simulink model "snap2_f_200msps_64i_4096c"  (R2019a)
settings: Solver=VariableStepDiscrete  StartTime=0.0  StopTime=10.0  RelTol=1e-3
undefined symbols (not defined in the file or in its folder): datetime, posixtime
libraries: xbsIndex_r4 x21354, casper_library_misc x297, casper_library_delays x19, xps_library x14, casper_library_sources x4
(part 4 of 217)

== system snap2_f_200msps_64i_4096c/delay ==
  note: counter starts at 1!!!
      | Simulation confirms this is the right
      | timing for the Serial -> Parallel converter to do The Right Thing
  sync : Inport
  din : Inport  Port=2
  65 : Subsystem  Commented=on
  Constant : xbsIndex_r4/Constant  const=2^max_delay_bits  gui_display_data_type=Fixed-point  arith_type=Unsigned  n_bits=32  bin_pt=0  preci_type=Single  exp_width=8  frac_width=24  explicit_period=on  period=1  equ=P=C  opselect=C  inp2=PCIN>>17  opr=+  inp1=P  carry=CIN  dbl_ovrd=off  block_type=constant
  Constant1 : xbsIndex_r4/Constant  Commented=on  const=0  gui_display_data_type=Fixed-point  arith_type=Unsigned  n_bits=32  bin_pt=0  preci_type=Single  exp_width=8  frac_width=24  explicit_period=on  period=1  equ=P=C  opselect=C  inp2=PCIN>>17  opr=+  inp1=P  carry=CIN  dbl_ovrd=off  block_type=constant
  Constant2 : xbsIndex_r4/Constant  Commented=on  const=0  gui_display_data_type=Boolean  arith_type=Boolean  n_bits=32  bin_pt=0  preci_type=Single  exp_width=8  frac_width=24  explicit_period=on  period=1  equ=P=C  opselect=C  inp2=PCIN>>17  opr=+  inp1=P  carry=CIN  dbl_ovrd=off  block_type=constant
  Counter : xbsIndex_r4/Counter  Commented=on  cnt_type=Free Running  cnt_to=Inf  operation=Up  start_count=1  cnt_by_val=1  arith_type=Unsigned  n_bits=6  bin_pt=0  load_pin=off  rst=off  en=off  explicit_period=on  period=1  use_behavioral_HDL=off  implementation=Fabric  dbl_ovrd=off  block_type=counter
  Delay : xbsIndex_r4/Delay  rst=off  infoeditControl=Selection of Reset will increase slice count due to use of real FFs and instead of SRLs  en=off  latency=7  reg_retiming=on  dbl_ovrd=off  block_type=delay
  Gateway Out{,1..7} (8 alike) : xbsIndex_r4/Gateway Out  Commented=on  inherit_from_input=off  hdl_port=off  rows=1  columns=1  UseAsDAC=off  DACChannel='1'  interface=None  automatic_assignment=on  address_offset=hex2dec('00')  intf_name=''  intf_description=''  timing_constraint=None  locs_specified=off  LOCs={}  io_standard={}  block_type=gatewayout
  Scope{,1..7} (8 alike) : Scope  Commented=on
  Serial to Parallel : xbsIndex_r4/Serial to Parallel  Commented=on  input_order=Most Significant Word First  arith_type=Unsigned  output_bits=13*64  bin_pt=0  rst=off  en=off  latency=1  dbl_ovrd=off  block_type=s2p
      settings: infoedit=Groups of samples presented serially at the input become single samples presented at the output.
  Slice : xbsIndex_r4/Slice  Commented=on  nbits=13  boolean_output=off  mode=Lower Bit Location + Width  bit1=0  base1=MSB of Input  bit0=0  base0=LSB of Input  dbl_ovrd=off  block_type=slice
  Slice1 : xbsIndex_r4/Slice  Commented=on  nbits=13  boolean_output=off  mode=Lower Bit Location + Width  bit1=0  base1=MSB of Input  bit0=0  base0=LSB of Input  dbl_ovrd=off  block_type=slice
  Slice2 : xbsIndex_r4/Slice  Commented=on  nbits=13  boolean_output=off  mode=Lower Bit Location + Width  bit1=0  base1=MSB of Input  bit0=13  base0=LSB of Input  dbl_ovrd=off  block_type=slice
  Slice3 : xbsIndex_r4/Slice  Commented=on  nbits=13  boolean_output=off  mode=Lower Bit Location + Width  bit1=0  base1=MSB of Input  bit0=13*2  base0=LSB of Input  dbl_ovrd=off  block_type=slice
  Subsystem : Subsystem
  Up Sample : xbsIndex_r4/Up Sample  Commented=on  sample_ratio=64  copy_samples=on  en=off  latency=1  dbl_ovrd=off  block_type=usamp
  bus_create : Subsystem  AncestorBlock=casper_library_flow_control/bus_create  mask(bus_create){inputNum=64}
      mask prompts: inputNum "Number of inputs:"
      mask init:
      | bus_create_init(gcb,...
      |     'inputNum', inputNum);
  bus_expand : Subsystem  AncestorBlock=casper_library_flow_control/bus_expand  mask(bus_expand){mode=divisions of equal size, outputNum=8*8, outputWidth=10, outputBinaryPt=0, outputArithmeticType=0, show_format=off, outputToWorkspace=off, variablePrefix=out, outputToModelAsWell=on}
      mask prompts: outputNum "Number of outputs:"; outputWidth "Output width:"; outputBinaryPt "Output binary point position:"; outputArithmeticType "Output arithmetic type (ufix=0, fix=1, bool=2):"; show_format "Print format string?"; outputToWorkspace "Output to workspace?"; variablePrefix "Variable name prefix:"; outputToModelAsWell "Output to model as well?"
      mask help:
      | Expands a 'bus' made using a bus_create or Xilinx
      | concat block.
      | The input will be divided into the specified number
      | of outputs with the specified arithmetic types.
      | Divisions are made from most significant bit.
      mask init: same as snap2_f_200msps_64i_4096c/autocorr/bus_expand
      settings: AttributesFormatString=64 outputs
      mask TypeOptions mode: divisions of equal size | divisions of arbitrary size
      mask Callback mode: bus_expand_callback();
      mask Callback outputWidth: bus_expand_callback();
      mask Callback outputToWorkspace: bus_expand_callback();
  bus_expand1 : Subsystem  AncestorBlock=casper_library_flow_control/bus_expand  mask(bus_expand){mode=divisions of equal size, outputNum=32, outputWidth=1, outputBinaryPt=0, outputArithmeticType=2, show_format=off, outputToWorkspace=off, variablePrefix=out, outputToModelAsWell=on}
      mask prompts: outputNum "Number of outputs:"; outputWidth "Output width:"; outputBinaryPt "Output binary point position:"; outputArithmeticType "Output arithmetic type (ufix=0, fix=1, bool=2):"; show_format "Print format string?"; outputToWorkspace "Output to workspace?"; variablePrefix "Variable name prefix:"; outputToModelAsWell "Output to model as well?"
      mask help:
      | Expands a 'bus' made using a bus_create or Xilinx
      | concat block.
      | The input will be divided into the specified number
      | of outputs with the specified arithmetic types.
      | Divisions are made from most significant bit.
      mask init: same as snap2_f_200msps_64i_4096c/autocorr/bus_expand
      settings: AttributesFormatString=32 outputs
      mask TypeOptions mode: divisions of equal size | divisions of arbitrary size
      mask Callback mode: bus_expand_callback();
      mask Callback outputWidth: bus_expand_callback();
      mask Callback outputToWorkspace: bus_expand_callback();
  bus_expand2 : Subsystem  AncestorBlock=casper_library_flow_control/bus_expand  mask(bus_expand){mode=divisions of equal size, outputNum=32, outputWidth=1, outputBinaryPt=0, outputArithmeticType=2, show_format=off, outputToWorkspace=off, variablePrefix=out, outputToModelAsWell=on}
      mask prompts: outputNum "Number of outputs:"; outputWidth "Output width:"; outputBinaryPt "Output binary point position:"; outputArithmeticType "Output arithmetic type (ufix=0, fix=1, bool=2):"; show_format "Print format string?"; outputToWorkspace "Output to workspace?"; variablePrefix "Variable name prefix:"; outputToModelAsWell "Output to model as well?"
      mask help:
      | Expands a 'bus' made using a bus_create or Xilinx
      | concat block.
      | The input will be divided into the specified number
      | of outputs with the specified arithmetic types.
      | Divisions are made from most significant bit.
      mask init: same as snap2_f_200msps_64i_4096c/autocorr/bus_expand
      settings: AttributesFormatString=32 outputs
      mask TypeOptions mode: divisions of equal size | divisions of arbitrary size
      mask Callback mode: bus_expand_callback();
      mask Callback outputWidth: bus_expand_callback();
      mask Callback outputToWorkspace: bus_expand_callback();
  delay0 : Subsystem  Tag=xps:sw_reg  AncestorBlock=xps_library/Memory/software_register  mask(swreg){io_dir=From Processor, io_delay=0, init_val=0, sample_period=1, names=reg, bitwidths=13, bin_pts=0, arith_types=0, sim_port=on, show_format=on, desc_str=""}
      mask prompts: io_dir "I/O direction"; io_delay "I/O delay"; init_val "Initial Value"; sample_period "Sample period"; names "Bitfield names [msb...lsb]"; bitwidths "Bitfield widths"; bin_pts "Bitfield binary pts"; arith_types "Bitfield types, ufix=0, fix=1, bool=2"; sim_port "Provide sim input/output?"; show_format "Print format string?"; desc_str "Description"
      mask help: A 32-bit software-accessible register. Can be divided into bitfields of varying widths and types using the fields in the block mask.
      mask init:
      | swreg_init(gcb)
      settings: AttributesFormatString=1input:uf13.0 = 13 bits
      mask TypeOptions io_dir: To Processor | From Processor
      mask Callback io_dir:
      | mask_enables = get_param(gcb, 'MaskEnables');
      | mask_names = get_param(gcb, 'MaskNames');
      | if strcmp(get_param(gcb, 'io_dir'), 'To Processor'),
      |     mask_enables{ismember(mask_names, 'sample_period')} = 'off';
      | else
      |     mask_enables{ismember(mask_names, 'sample_period')} = 'on';
      | end
      | set_param(gcb, 'MaskEnables', mask_enables);
      mask DialogControl ParameterTabVar0 Prompt: Setup
  delay1 : Subsystem  Tag=xps:sw_reg  AncestorBlock=xps_library/Memory/software_register  mask(swreg){io_dir=From Processor, io_delay=0, init_val=0, sample_period=1, names=reg, bitwidths=13, bin_pts=0, arith_types=0, sim_port=on, show_format=on, desc_str=""}
      mask prompts: io_dir "I/O direction"; io_delay "I/O delay"; init_val "Initial Value"; sample_period "Sample period"; names "Bitfield names [msb...lsb]"; bitwidths "Bitfield widths"; bin_pts "Bitfield binary pts"; arith_types "Bitfield types, ufix=0, fix=1, bool=2"; sim_port "Provide sim input/output?"; show_format "Print format string?"; desc_str "Description"
      mask help: A 32-bit software-accessible register. Can be divided into bitfields of varying widths and types using the fields in the block mask.
      mask init:
      | swreg_init(gcb)
      settings: AttributesFormatString=1input:uf13.0 = 13 bits
      mask TypeOptions io_dir: To Processor | From Processor
      mask Callback io_dir:
      | mask_enables = get_param(gcb, 'MaskEnables');
      | mask_names = get_param(gcb, 'MaskNames');
      | if strcmp(get_param(gcb, 'io_dir'), 'To Processor'),
      |     mask_enables{ismember(mask_names, 'sample_period')} = 'off';
      | else
      |     mask_enables{ismember(mask_names, 'sample_period')} = 'on';
      | end
      | set_param(gcb, 'MaskEnables', mask_enables);
      mask DialogControl ParameterTabVar0 Prompt: Setup
  delay_en0 : Subsystem  Tag=xps:sw_reg  AncestorBlock=xps_library/Memory/software_register  mask(swreg){io_dir=From Processor, io_delay=0, init_val=0, sample_period=1, names=reg, bitwidths=32, bin_pts=0, arith_types=0, sim_port=on, show_format=on, desc_str=""}
      mask prompts: io_dir "I/O direction"; io_delay "I/O delay"; init_val "Initial Value"; sample_period "Sample period"; names "Bitfield names [msb...lsb]"; bitwidths "Bitfield widths"; bin_pts "Bitfield binary pts"; arith_types "Bitfield types, ufix=0, fix=1, bool=2"; sim_port "Provide sim input/output?"; show_format "Print format string?"; desc_str "Description"
      mask help: A 32-bit software-accessible register. Can be divided into bitfields of varying widths and types using the fields in the block mask.
      mask init:
      | swreg_init(gcb)
      settings: AttributesFormatString=1input:uf32.0 = 32 bits
      mask TypeOptions io_dir: To Processor | From Processor
      mask Callback io_dir:
      | mask_enables = get_param(gcb, 'MaskEnables');
      | mask_names = get_param(gcb, 'MaskNames');
      | if strcmp(get_param(gcb, 'io_dir'), 'To Processor'),
      |     mask_enables{ismember(mask_names, 'sample_period')} = 'off';
      | else
      |     mask_enables{ismember(mask_names, 'sample_period')} = 'on';
      | end
      | set_param(gcb, 'MaskEnables', mask_enables);
      mask DialogControl ParameterTabVar0 Prompt: Setup
  delay_en1 : Subsystem  Tag=xps:sw_reg  AncestorBlock=xps_library/Memory/software_register  mask(swreg){io_dir=From Processor, io_delay=0, init_val=0, sample_period=1, names=reg, bitwidths=32, bin_pts=0, arith_types=0, sim_port=on, show_format=on, desc_str=""}
      mask prompts: io_dir "I/O direction"; io_delay "I/O delay"; init_val "Initial Value"; sample_period "Sample period"; names "Bitfield names [msb...lsb]"; bitwidths "Bitfield widths"; bin_pts "Bitfield binary pts"; arith_types "Bitfield types, ufix=0, fix=1, bool=2"; sim_port "Provide sim input/output?"; show_format "Print format string?"; desc_str "Description"
      mask help: A 32-bit software-accessible register. Can be divided into bitfields of varying widths and types using the fields in the block mask.
      mask init:
      | swreg_init(gcb)
      settings: AttributesFormatString=1input:uf32.0 = 32 bits
      mask TypeOptions io_dir: To Processor | From Processor
      mask Callback io_dir:
      | mask_enables = get_param(gcb, 'MaskEnables');
      | mask_names = get_param(gcb, 'MaskNames');
      | if strcmp(get_param(gcb, 'io_dir'), 'To Processor'),
      |     mask_enables{ismember(mask_names, 'sample_period')} = 'off';
      | else
      |     mask_enables{ismember(mask_names, 'sample_period')} = 'on';
      | end
      | set_param(gcb, 'MaskEnables', mask_enables);
      mask DialogControl ParameterTabVar0 Prompt: Setup
  delay_store0 : Subsystem
  delay_store1 : Subsystem
  delays : Subsystem  Tag=xps:bram  Commented=on  AncestorBlock=xps_library/Memory/shared_bram  mask{sample_rate=1, init_vals=[0:2^6-1], data_bin_pt=0, optimization=Minimum_Area, reg_core_output=off, reg_prim_output=off, data_width=32, addr_width=6, arith_type=Unsigned, desc_str="", type_desc=""}
      mask prompts: sample_rate "Sample rate"; init_vals "Initial values (simulation only)"; data_bin_pt "Data Binary Point"; reg_core_output "Register Core Output"; reg_prim_output "Register Primitive Output"; data_width "Data Width"; addr_width "Address width"; arith_type "Output Data Type"; desc_str "Description"; type_desc "Word Type Description"
      mask init:
      | shared_bram_mask;
      mask TypeOptions optimization: Minimum_Area | Low_Power
      mask TypeOptions data_width: 8 | 16 | 32 | 64 | 128
      mask TypeOptions arith_type: Unsigned | Signed  (2's comp)
      mask DialogControl Container4 Prompt: Configuration
      mask DialogControl Container10 Prompt: Documentation
  max_delay : Subsystem  Tag=xps:sw_reg  AncestorBlock=xps_library/Memory/software_register  mask(swreg){io_dir=To Processor, io_delay=0, init_val=0, sample_period=1, names=reg, bitwidths=32, bin_pts=0, arith_types=0, sim_port=on, show_format=off, desc_str=|}
      mask desc_str=|
      | Interpretted as a unint32 value, contains the maximum
      | allowed delay, in ADC samples, which may be applied
      | to a data stream.
      mask prompts: io_dir "I/O direction"; io_delay "I/O delay"; init_val "Initial Value"; sample_period "Sample period"; names "Bitfield names [msb...lsb]"; bitwidths "Bitfield widths"; bin_pts "Bitfield binary pts"; arith_types "Bitfield types, ufix=0, fix=1, bool=2"; sim_port "Provide sim input/output?"; show_format "Print format string?"; desc_str "Description"
      mask help: A 32-bit software-accessible register. Can be divided into bitfields of varying widths and types using the fields in the block mask.
      mask init:
      | swreg_init(gcb)
      settings: AttributesFormatString=1output
      mask TypeOptions io_dir: To Processor | From Processor
      mask Callback io_dir:
      | mask_enables = get_param(gcb, 'MaskEnables');
      | mask_names = get_param(gcb, 'MaskNames');
      | if strcmp(get_param(gcb, 'io_dir'), 'To Processor'),
      |     mask_enables{ismember(mask_names, 'sample_period')} = 'off';
      | else
      |     mask_enables{ismember(mask_names, 'sample_period')} = 'on';
      | end
      | set_param(gcb, 'MaskEnables', mask_enables);
      mask DialogControl ParameterTabVar0 Prompt: Setup
  sync_out : Outport
  dout : Outport  Port=2
  wires:
  sync/1 -> Delay/1
  din/1 -> bus_expand/1(bus_in)
  bus_create/1(bus_out) -> dout/1
  Constant/1 -> max_delay/1(out_reg)
  Delay/1 -> sync_out/1
  Counter/1 -> delays/1(addr)
  Constant1/1 -> delays/2(data_in)
  Constant2/1 -> delays/3(we)
  delays/1(data_out) -> Slice/1
  Serial to Parallel/1 -> Up Sample/1, Slice3/1, Slice2/1, Slice1/1
  Slice/1 -> Gateway Out/1, Serial to Parallel/1
  Subsystem/1(Out1) -> bus_create/1(in1)
  Subsystem/2(Out2) -> bus_create/2(in2)
  Subsystem/3(Out3) -> bus_create/3(in3)
  Subsystem/4(Out4) -> bus_create/4(in4)
  Subsystem/5(Out5) -> bus_create/5(in5)
  Subsystem/6(Out6) -> bus_create/6(in6)
  Subsystem/7(Out7) -> bus_create/7(in7)
  Subsystem/8(Out8) -> bus_create/8(in8)
  Subsystem/9(Out9) -> bus_create/9(in9)
  Subsystem/10(Out10) -> bus_create/10(in10)
  Subsystem/11(Out11) -> bus_create/11(in11)
  Subsystem/12(Out12) -> bus_create/12(in12)
  Subsystem/13(Out13) -> bus_create/13(in13)
  Subsystem/14(Out14) -> bus_create/14(in14)
  Subsystem/15(Out15) -> bus_create/15(in15)
  Subsystem/16(Out16) -> bus_create/16(in16)
  Subsystem/17(Out17) -> bus_create/17(in17)
  Subsystem/18(Out18) -> bus_create/18(in18)
  Subsystem/19(Out19) -> bus_create/19(in19)
  Subsystem/20(Out20) -> bus_create/20(in20)
  Subsystem/21(Out21) -> bus_create/21(in21)
  Subsystem/22(Out22) -> bus_create/22(in22)
  Subsystem/23(Out23) -> bus_create/23(in23)
  Subsystem/24(Out24) -> bus_create/24(in24)
  Subsystem/25(Out25) -> bus_create/25(in25)
  Subsystem/26(Out26) -> bus_create/26(in26)
  Subsystem/27(Out27) -> bus_create/27(in27)
  Subsystem/28(Out28) -> bus_create/28(in28)
  Subsystem/29(Out29) -> bus_create/29(in29)
  Subsystem/30(Out30) -> bus_create/30(in30)
  Subsystem/31(Out31) -> bus_create/31(in31)
  Subsystem/32(Out32) -> bus_create/32(in32)
  Subsystem/33(Out33) -> bus_create/33(in33)
  Subsystem/34(Out34) -> bus_create/34(in34)
  Subsystem/35(Out35) -> bus_create/35(in35)
  Subsystem/36(Out36) -> bus_create/36(in36)
  Subsystem/37(Out37) -> bus_create/37(in37)
  Subsystem/38(Out38) -> bus_create/38(in38)
  Subsystem/39(Out39) -> bus_create/39(in39)
  Subsystem/40(Out40) -> bus_create/40(in40)
  Subsystem/41(Out41) -> bus_create/41(in41)
  Subsystem/42(Out42) -> bus_create/42(in42)
  Subsystem/43(Out43) -> bus_create/43(in43)
  Subsystem/44(Out44) -> bus_create/44(in44)
  Subsystem/45(Out45) -> bus_create/45(in45)
  Subsystem/46(Out46) -> bus_create/46(in46)
  Subsystem/47(Out47) -> bus_create/47(in47)
  Subsystem/48(Out48) -> bus_create/48(in48)
  Subsystem/49(Out49) -> bus_create/49(in49)
  Subsystem/50(Out50) -> bus_create/50(in50)
  Subsystem/51(Out51) -> bus_create/51(in51)
  Subsystem/52(Out52) -> bus_create/52(in52)
  Subsystem/53(Out53) -> bus_create/53(in53)
  Subsystem/54(Out54) -> bus_create/54(in54)
  Subsystem/55(Out55) -> bus_create/55(in55)
  Subsystem/56(Out56) -> bus_create/56(in56)
  Subsystem/57(Out57) -> bus_create/57(in57)
  Subsystem/58(Out58) -> bus_create/58(in58)
  Subsystem/59(Out59) -> bus_create/59(in59)
  Subsystem/60(Out60) -> bus_create/60(in60)
  Subsystem/61(Out61) -> bus_create/61(in61)
  Subsystem/62(Out62) -> bus_create/62(in62)
  Subsystem/63(Out63) -> bus_create/63(in63)
  Subsystem/64(Out64) -> bus_create/64(in64)
  bus_expand/1(msb_out64) -> Subsystem/1(In1)
  bus_expand/2(out63) -> Subsystem/2(In3)
  bus_expand/3(out62) -> Subsystem/3(In2)
  bus_expand/4(out61) -> Subsystem/4(In4)
  bus_expand/5(out60) -> Subsystem/5(In5)
  bus_expand/6(out59) -> Subsystem/6(In6)
  bus_expand/7(out58) -> Subsystem/7(In7)
  bus_expand/8(out57) -> Subsystem/8(In8)
  bus_expand/9(out56) -> Subsystem/9(In9)
  bus_expand/10(out55) -> Subsystem/10(In10)
  bus_expand/11(out54) -> Subsystem/11(In11)
  bus_expand/12(out53) -> Subsystem/12(In12)
  bus_expand/13(out52) -> Subsystem/13(In13)
  bus_expand/14(out51) -> Subsystem/14(In14)
  bus_expand/15(out50) -> Subsystem/15(In15)
  bus_expand/16(out49) -> Subsystem/16(In16)
  bus_expand/17(out48) -> Subsystem/17(In17)
  bus_expand/18(out47) -> Subsystem/18(In18)
  bus_expand/19(out46) -> Subsystem/19(In19)
  bus_expand/20(out45) -> Subsystem/20(In20)
  bus_expand/21(out44) -> Subsystem/21(In21)
  bus_expand/22(out43) -> Subsystem/22(In22)
  bus_expand/23(out42) -> Subsystem/23(In23)
  bus_expand/24(out41) -> Subsystem/24(In24)
  bus_expand/25(out40) -> Subsystem/25(In25)
  bus_expand/26(out39) -> Subsystem/26(In26)
  bus_expand/27(out38) -> Subsystem/27(In27)
  bus_expand/28(out37) -> Subsystem/28(In28)
  bus_expand/29(out36) -> Subsystem/29(In29)
  bus_expand/30(out35) -> Subsystem/30(In30)
  bus_expand/31(out34) -> Subsystem/31(In31)
  bus_expand/32(out33) -> Subsystem/32(In32)
  bus_expand/33(out32) -> Subsystem/33(In33)
  bus_expand/34(out31) -> Subsystem/34(In34)
  bus_expand/35(out30) -> Subsystem/35(In35)
  bus_expand/36(out29) -> Subsystem/36(In36)
  bus_expand/37(out28) -> Subsystem/37(In37)
  bus_expand/38(out27) -> Subsystem/38(In38)
  bus_expand/39(out26) -> Subsystem/39(In39)
  bus_expand/40(out25) -> Subsystem/40(In40)
  bus_expand/41(out24) -> Subsystem/41(In41)
  bus_expand/42(out23) -> Subsystem/42(In42)
  bus_expand/43(out22) -> Subsystem/43(In43)
  bus_expand/44(out21) -> Subsystem/44(In44)
  bus_expand/45(out20) -> Subsystem/45(In45)
  bus_expand/46(out19) -> Subsystem/46(In46)
  bus_expand/47(out18) -> Subsystem/47(In47)
  bus_expand/48(out17) -> Subsystem/48(In48)
  bus_expand/49(out16) -> Subsystem/49(In49)
  bus_expand/50(out15) -> Subsystem/50(In50)
  bus_expand/51(out14) -> Subsystem/51(In51)
  bus_expand/52(out13) -> Subsystem/52(In52)
  bus_expand/53(out12) -> Subsystem/53(In53)
  bus_expand/54(out11) -> Subsystem/54(In54)
  bus_expand/55(out10) -> Subsystem/55(In55)
  bus_expand/56(out9) -> Subsystem/56(In56)
  bus_expand/57(out8) -> Subsystem/57(In57)
  bus_expand/58(out7) -> Subsystem/58(In58)
  bus_expand/59(out6) -> Subsystem/59(In59)
  bus_expand/60(out5) -> Subsystem/60(In60)
  bus_expand/61(out4) -> Subsystem/61(In61)
  bus_expand/62(out3) -> Subsystem/62(In62)
  bus_expand/63(out2) -> Subsystem/63(In63)
  bus_expand/64(lsb_out1) -> Subsystem/64(In64)
  Gateway Out/1 -> Scope/1
  Gateway Out1/1 -> Scope1/1
  Gateway Out2/1 -> Scope2/1
  Gateway Out3/1 -> Scope3/1
  Slice1/1 -> Gateway Out3/1
  Slice2/1 -> Gateway Out4/1
  Gateway Out4/1 -> Scope4/1
  Gateway Out5/1 -> Scope5/1
  Slice3/1 -> Gateway Out5/1
  Gateway Out7/1 -> Scope7/1
  Gateway Out6/1 -> Scope6/1
  delay0/1(in_reg) -> delay_store0/1(delay_in)
  delay_store0/1(delay0) -> Subsystem/65(delay1)
  delay_store0/2(delay1) -> Subsystem/66(delay2)
  delay_store0/3(delay2) -> Subsystem/67(delay3)
  delay_store0/4(delay3) -> Subsystem/68(delay4)
  delay_store0/5(delay4) -> Subsystem/69(delay5)
  delay_store0/6(delay5) -> Subsystem/70(delay6)
  delay_store0/7(delay6) -> Subsystem/71(delay7)
  delay_store0/8(delay7) -> Subsystem/72(delay8)
  delay_store0/9(delay8) -> Subsystem/73(delay9)
  delay_store0/10(delay9) -> Subsystem/74(delay10)
  delay_store0/11(delay10) -> Subsystem/75(delay11)
  delay_store0/12(delay11) -> Subsystem/76(delay12)
  delay_store0/13(delay12) -> Subsystem/77(delay13)
  delay_store0/14(delay13) -> Subsystem/78(delay14)
  delay_store0/15(delay14) -> Subsystem/79(delay15)
  delay_store0/16(delay15) -> Subsystem/80(delay16)
  delay_store0/17(delay16) -> Subsystem/81(delay17)
  delay_store0/18(delay17) -> Subsystem/82(delay18)
  delay_store0/19(delay18) -> Subsystem/83(delay19)
  delay_store0/20(delay19) -> Subsystem/84(delay20)
  delay_store0/21(delay20) -> Subsystem/85(delay21)
  delay_store0/22(delay21) -> Subsystem/86(delay22)
  delay_store0/23(delay22) -> Subsystem/87(delay23)
  delay_store0/24(delay23) -> Subsystem/88(delay24)
  delay_store0/25(delay24) -> Subsystem/89(delay25)
  delay_store0/26(delay25) -> Subsystem/90(delay26)
  delay_store0/27(delay26) -> Subsystem/91(delay27)
  delay_store0/28(delay27) -> Subsystem/92(delay28)
  delay_store0/29(delay28) -> Subsystem/93(delay29)
  delay_store0/30(delay29) -> Subsystem/94(delay30)
  delay_store0/31(delay30) -> Subsystem/95(delay31)
  delay_store0/32(delay31) -> Subsystem/96(delay32)
  delay_store1/1(delay0) -> Subsystem/97(delay33)
  delay_store1/2(delay1) -> Subsystem/98(delay34)
  delay_store1/3(delay2) -> Subsystem/99(delay35)
  delay_store1/4(delay3) -> Subsystem/100(delay36)
  delay_store1/5(delay4) -> Subsystem/101(delay37)
  delay_store1/6(delay5) -> Subsystem/102(delay38)
  delay_store1/7(delay6) -> Subsystem/103(delay39)
  delay_store1/8(delay7) -> Subsystem/104(delay40)
  delay_store1/9(delay8) -> Subsystem/105(delay41)
  delay_store1/10(delay9) -> Subsystem/106(delay42)
  delay_store1/11(delay10) -> Subsystem/107(delay43)
  delay_store1/12(delay11) -> Subsystem/108(delay44)
  delay_store1/13(delay12) -> Subsystem/109(delay45)
  delay_store1/14(delay13) -> Subsystem/110(delay46)
  delay_store1/15(delay14) -> Subsystem/111(delay47)
  delay_store1/16(delay15) -> Subsystem/112(delay48)
  delay_store1/17(delay16) -> Subsystem/113(delay49)
  delay_store1/18(delay17) -> Subsystem/114(delay50)
  delay_store1/19(delay18) -> Subsystem/115(delay51)
  delay_store1/20(delay19) -> Subsystem/116(delay52)
  delay_store1/21(delay20) -> Subsystem/117(delay53)
  delay_store1/22(delay21) -> Subsystem/118(delay54)
  delay_store1/23(delay22) -> Subsystem/119(delay55)
  delay_store1/24(delay23) -> Subsystem/120(delay56)
  delay_store1/25(delay24) -> Subsystem/121(delay57)
  delay_store1/26(delay25) -> Subsystem/122(delay58)
  delay_store1/27(delay26) -> Subsystem/123(delay59)
  delay_store1/28(delay27) -> Subsystem/124(delay60)
  delay_store1/29(delay28) -> Subsystem/125(delay61)
  delay_store1/30(delay29) -> Subsystem/126(delay62)
  delay_store1/31(delay30) -> Subsystem/127(delay63)
  delay_store1/32(delay31) -> Subsystem/128(delay64)
  bus_expand1/1(msb_out32) -> delay_store0/2(en0)
  bus_expand1/2(out31) -> delay_store0/3(en1)
  bus_expand1/3(out30) -> delay_store0/4(en2)
  bus_expand1/4(out29) -> delay_store0/5(en3)
  bus_expand1/5(out28) -> delay_store0/6(en4)
  bus_expand1/6(out27) -> delay_store0/7(en5)
  bus_expand1/7(out26) -> delay_store0/8(en6)
  bus_expand1/8(out25) -> delay_store0/9(en7)
  bus_expand1/9(out24) -> delay_store0/10(en8)
  bus_expand1/10(out23) -> delay_store0/11(en9)
  bus_expand1/11(out22) -> delay_store0/12(en10)
  bus_expand1/12(out21) -> delay_store0/13(en11)
  bus_expand1/13(out20) -> delay_store0/14(en12)
  bus_expand1/14(out19) -> delay_store0/15(en13)
  bus_expand1/15(out18) -> delay_store0/16(en14)
  bus_expand1/16(out17) -> delay_store0/17(en15)
  bus_expand1/17(out16) -> delay_store0/18(en16)
  bus_expand1/18(out15) -> delay_store0/19(en17)
  bus_expand1/19(out14) -> delay_store0/20(en18)
  bus_expand1/20(out13) -> delay_store0/21(en19)
  bus_expand1/21(out12) -> delay_store0/22(en20)
  bus_expand1/22(out11) -> delay_store0/23(en21)
  bus_expand1/23(out10) -> delay_store0/24(en22)
  bus_expand1/24(out9) -> delay_store0/25(en23)
  bus_expand1/25(out8) -> delay_store0/26(en24)
  bus_expand1/26(out7) -> delay_store0/27(en25)
  bus_expand1/27(out6) -> delay_store0/28(en26)
  bus_expand1/28(out5) -> delay_store0/29(en27)
  bus_expand1/29(out4) -> delay_store0/30(en28)
  bus_expand1/30(out3) -> delay_store0/31(en29)
  bus_expand1/31(out2) -> delay_store0/32(en30)
  bus_expand1/32(lsb_out1) -> delay_store0/33(en31)
  delay_en0/1(in_reg) -> bus_expand1/1(bus_in)
  delay_en1/1(in_reg) -> bus_expand2/1(bus_in)
  delay1/1(in_reg) -> delay_store1/1(delay_in)
  bus_expand2/1(msb_out32) -> delay_store1/2(en0)
  bus_expand2/2(out31) -> delay_store1/3(en1)
  bus_expand2/3(out30) -> delay_store1/4(en2)
  bus_expand2/4(out29) -> delay_store1/5(en3)
  bus_expand2/5(out28) -> delay_store1/6(en4)
  bus_expand2/6(out27) -> delay_store1/7(en5)
  bus_expand2/7(out26) -> delay_store1/8(en6)
  bus_expand2/8(out25) -> delay_store1/9(en7)
  bus_expand2/9(out24) -> delay_store1/10(en8)
  bus_expand2/10(out23) -> delay_store1/11(en9)
  bus_expand2/11(out22) -> delay_store1/12(en10)
  bus_expand2/12(out21) -> delay_store1/13(en11)
  bus_expand2/13(out20) -> delay_store1/14(en12)
  bus_expand2/14(out19) -> delay_store1/15(en13)
  bus_expand2/15(out18) -> delay_store1/16(en14)
  bus_expand2/16(out17) -> delay_store1/17(en15)
  bus_expand2/17(out16) -> delay_store1/18(en16)
  bus_expand2/18(out15) -> delay_store1/19(en17)
  bus_expand2/19(out14) -> delay_store1/20(en18)
  bus_expand2/20(out13) -> delay_store1/21(en19)
  bus_expand2/21(out12) -> delay_store1/22(en20)
  bus_expand2/22(out11) -> delay_store1/23(en21)
  bus_expand2/23(out10) -> delay_store1/24(en22)
  bus_expand2/24(out9) -> delay_store1/25(en23)
  bus_expand2/25(out8) -> delay_store1/26(en24)
  bus_expand2/26(out7) -> delay_store1/27(en25)
  bus_expand2/27(out6) -> delay_store1/28(en26)
  bus_expand2/28(out5) -> delay_store1/29(en27)
  bus_expand2/29(out4) -> delay_store1/30(en28)
  bus_expand2/30(out3) -> delay_store1/31(en29)
  bus_expand2/31(out2) -> delay_store1/32(en30)
  bus_expand2/32(lsb_out1) -> delay_store1/33(en31)

== system snap2_f_200msps_64i_4096c/eq ==
  sync : Inport
  din : Inport  Port=2
  bus_create2 : Subsystem  AncestorBlock=casper_library_flow_control/bus_create  mask(bus_create){inputNum=4}
      mask prompts: inputNum "Number of inputs:"
      mask init:
      | bus_create_init(gcb,...
      |     'inputNum', inputNum);
  bus_expand4 : Subsystem  AncestorBlock=casper_library_flow_control/bus_expand  mask(bus_expand){mode=divisions of equal size, outputNum=4, outputWidth=36*8, outputBinaryPt=0, outputArithmeticType=0, show_format=off, outputToWorkspace=off, variablePrefix=out, outputToModelAsWell=on}
      mask prompts: outputNum "Number of outputs:"; outputWidth "Output width:"; outputBinaryPt "Output binary point position:"; outputArithmeticType "Output arithmetic type (ufix=0, fix=1, bool=2):"; show_format "Print format string?"; outputToWorkspace "Output to workspace?"; variablePrefix "Variable name prefix:"; outputToModelAsWell "Output to model as well?"
      mask help:
      | Expands a 'bus' made using a bus_create or Xilinx
      | concat block.
      | The input will be divided into the specified number
      | of outputs with the specified arithmetic types.
      | Divisions are made from most significant bit.
      mask init: same as snap2_f_200msps_64i_4096c/autocorr/bus_expand
      settings: AttributesFormatString=4 outputs
      mask TypeOptions mode: divisions of equal size | divisions of arbitrary size
      mask Callback mode: bus_expand_callback();
      mask Callback outputWidth: bus_expand_callback();
      mask Callback outputToWorkspace: bus_expand_callback();
  core0 : Subsystem  mask{nchan=12-3, nants=16, n_bp=2}
      mask prompts: nchan "Number of fft channels (2^?)"; nants "Number of Antennas"; n_bp "Coefficient binary point position"
  core1 : Subsystem  mask{nchan=12-3, nants=16, n_bp=2}
      mask prompts: nchan "Number of fft channels (2^?)"; nants "Number of Antennas"; n_bp "Coefficient binary point position"
  core2 : Subsystem  mask{nchan=12-3, nants=16, n_bp=2}
      mask prompts: nchan "Number of fft channels (2^?)"; nants "Number of Antennas"; n_bp "Coefficient binary point position"
  core3 : Subsystem  mask{nchan=12-3, nants=16, n_bp=2}
      mask prompts: nchan "Number of fft channels (2^?)"; nants "Number of Antennas"; n_bp "Coefficient binary point position"
  sync_out : Outport
  dout : Outport  Port=2
  wires:
  core0/1(sync_out) -> sync_out/1
  din/1 -> bus_expand4/1(bus_in)
  sync/1 -> [sync_in]
  [sync_in] -> core0/1(sync)
  [sync_in] -> core1/1(sync)
  [sync_in] -> core2/1(sync)
  [sync_in] -> core3/1(sync)
  bus_expand4/1(msb_out4) -> core0/2(in)
  bus_expand4/2(out3) -> core1/2(in)
  bus_expand4/3(out2) -> core2/2(in)
  bus_expand4/4(lsb_out1) -> core3/2(in)
  core1/1(sync_out) -> ?
  core2/1(sync_out) -> ?
  core3/1(sync_out) -> ?
  core1/2(dout) -> bus_create2/2(in2)
  core2/2(dout) -> bus_create2/3(in3)
  core0/2(dout) -> bus_create2/1(in1)
  core3/2(dout) -> bus_create2/4(in4)
  bus_create2/1(bus_out) -> dout/1

== system snap2_f_200msps_64i_4096c/eth ==
  note: bit 19
  note: bit 18
  note: bit 1
  note: bit 0
  note: only allow enable
      | state to change at the end
      | of a packet.
      |
      | This avoids overflows arising
      | from part of a packet being
      | clocked in to the core
      | but the EOF being disable
  data : Inport
  vld : Inport  Port=2
  eof : Inport  Port=3
  dest_ip : Inport  Port=4
  port : Inport  Port=5
  Constant : xbsIndex_r4/Constant  const=0  gui_display_data_type=Boolean  arith_type=Boolean  n_bits=1  bin_pt=0  preci_type=Single  exp_width=8  frac_width=24  explicit_period=on  period=1  equ=P=C  opselect=C  inp2=PCIN>>17  opr=+  inp1=P  carry=CIN  dbl_ovrd=off  block_type=constant
  Constant1 : xbsIndex_r4/Constant  const=0  gui_display_data_type=Boolean  arith_type=Boolean  n_bits=1  bin_pt=0  preci_type=Single  exp_width=8  frac_width=24  explicit_period=on  period=1  equ=P=C  opselect=C  inp2=PCIN>>17  opr=+  inp1=P  carry=CIN  dbl_ovrd=off  block_type=constant
  Delay{5..11} (7 alike) : xbsIndex_r4/Delay  rst=off  infoeditControl=Selection of Reset will increase slice count due to use of real FFs and instead of SRLs  en=off  latency=1  reg_retiming=off  dbl_ovrd=off  block_type=delay
  Logical : xbsIndex_r4/Logical  logical_function=AND  inputs=2  en=off  latency=0  precision=Full  arith_type=Unsigned  n_bits=16  bin_pt=0  align_bp=on  dbl_ovrd=off  block_type=logical
  Logical1 : xbsIndex_r4/Logical  logical_function=OR  inputs=2  en=off  latency=0  precision=Full  arith_type=Unsigned  n_bits=16  bin_pt=0  align_bp=on  dbl_ovrd=off  block_type=logical
  Register : xbsIndex_r4/Register  init=0  rst=off  en=on  dbl_ovrd=off  block_type=register
  Slice : xbsIndex_r4/Slice  nbits=1  boolean_output=on  mode=Lower Bit Location + Width  bit1=0  base1=MSB of Input  bit0=0  base0=LSB of Input  dbl_ovrd=off  block_type=slice
  Slice1 : xbsIndex_r4/Slice  nbits=1  boolean_output=on  mode=Lower Bit Location + Width  bit1=0  base1=MSB of Input  bit0=1  base0=LSB of Input  dbl_ovrd=off  block_type=slice
  Slice3 : xbsIndex_r4/Slice  nbits=1  boolean_output=on  mode=Lower Bit Location + Width  bit1=0  base1=MSB of Input  bit0=2+16  base0=LSB of Input  dbl_ovrd=off  block_type=slice
  Slice4 : xbsIndex_r4/Slice  nbits=1  boolean_output=on  mode=Lower Bit Location + Width  bit1=0  base1=MSB of Input  bit0=3+16  base0=LSB of Input  dbl_ovrd=off  block_type=slice
  ctrl : Subsystem  Tag=xps:sw_reg  AncestorBlock=xps_library/Memory/software_register  mask(swreg){io_dir=From Processor, io_delay=0, init_val=0, sample_period=1, names=reg, bitwidths=32, bin_pts=0, arith_types=0, sim_port=on, show_format=off, desc_str=|}
      mask desc_str=|
      | 40GbE control register. Bit ``0`` is an active high reset
      | of the 40GbE interface core. Bit ``1`` is an active
      | high transmission enable for the core, which takes
      | effect either after the next packet is sent, or when
      | the ``force`` flag is asserted. Bit ``18`` is
      | an active high reset for statistics provided by the
      | Ethernet core. Bit ``19`` is an active high ``force``
      | signal, which causes the current transmission enable
      | flag to immediately take effect.
      mask prompts: io_dir "I/O direction"; io_delay "I/O delay"; init_val "Initial Value"; sample_period "Sample period"; names "Bitfield names [msb...lsb]"; bitwidths "Bitfield widths"; bin_pts "Bitfield binary pts"; arith_types "Bitfield types, ufix=0, fix=1, bool=2"; sim_port "Provide sim input/output?"; show_format "Print format string?"; desc_str "Description"
      mask help: A 32-bit software-accessible register. Can be divided into bitfields of varying widths and types using the fields in the block mask.
      mask init:
      | swreg_init(gcb)
      settings: AttributesFormatString=1input
      mask TypeOptions io_dir: To Processor | From Processor
      mask Callback io_dir:
      | mask_enables = get_param(gcb, 'MaskEnables');
      | mask_names = get_param(gcb, 'MaskNames');
      | if strcmp(get_param(gcb, 'io_dir'), 'To Processor'),
      |     mask_enables{ismember(mask_names, 'sample_period')} = 'off';
      | else
      |     mask_enables{ismember(mask_names, 'sample_period')} = 'on';
      | end
      | set_param(gcb, 'MaskEnables', mask_enables);
      mask DialogControl ParameterTabVar0 Prompt: Setup
  forty_gbe : Subsystem  Tag=xps:forty_gbe  AncestorBlock=xps_library/IO/forty_gbe  InitFcn=forty_gbe_init  mask(forty_gbe){flavour=cx4, slot=1, port_r1=0, port_r2_cx4=0, port_r2_sfpp=0, port=0, rx_dist_ram=on, large_frames=on, input_pipeline_delay=0, show_param=on, pre_emph_r2=0.74, pre_emph=3, post_emph_r2=0.18, rxeqmix_r2=7, swing_r2=940, swing=800, fab_en=on, fab_mac=hex2dec('123456780000'), fab_ip=192*(2^24) + 168*(2^16) + 5*(2^8) + 20*(2^0), fab_udp=10000, fab_gate=1, cpu_rx_en=off, cpu_tx_en=off, ttl=hex2dec('FF'), promisc_mode=off, debug_ctr_width=32, debug_en_all=off, debug_dis_all=off, txctr=on, txerrctr=off, txerrctr_len=100, txofctr=on, txfullctr=on, txvldctr=on, txsnaplen=0 - no snap, rxctr=off, rxerrctr=off, rxerrctr_len=100, rxofctr=off, rxbadctr=off, rxvldctr=off, rxeofctr=off, rxsnaplen=0 - no snap, rxsrcip=off, rxdstip=off}
      mask prompts: flavour "Mezzanine card flavour"; slot "Card slot"; port_r1 "Port"; port_r2_cx4 "Port"; port_r2_sfpp "Port"; rx_dist_ram "Shallow RX Fifo (Beware overruns!)"; large_frames "Enable Large TX Frames (8k+512)"; input_pipeline_delay "Incoming pipeline delay"; show_param "---------------------- Show Implementation Parameters -----------------------------------------------------------------------------------"; pre_emph_r2 "Pre-emphasis (dB)"; pre_emph "Pre-emphasis"; post_emph_r2 "Post-emphasis (dB)"; rxeqmix_r2 "Receive equalisation"; swing_r2 "Driver Swing Control (mVppd)"; swing "Differential swing"; fab_en "Enable fabric on startup"; fab_mac "Fabric MAC Address"; fab_ip "Fabric IP Address"; fab_udp "Fabric UDP Port"; fab_gate "Fabric Gateway"; cpu_rx_en "Enable CPU RX"; cpu_tx_en "Enable CPU TX"; promisc_mode "Promiscuous mode"; debug_ctr_width "Debug counter width"; debug_en_all "Enable all counters (overrides individual settings)"; debug_dis_all "Disable all counters (overrides individual settings)"; txctr "TX - core_txctr"; txerrctr "TX packet length error - core_txerrctr"; txerrctr_len "-- expected TX packet length"; txofctr "TX overflow - core_txofctr"; txfullctr "TX full - core_txfullctr"; txvldctr "TX valid cycle - core_txvldctr"; txsnaplen "TX snapshot length"; rxctr "RX - core_rxctr"; rxerrctr "RX packet length error - core_rxerrctr"; rxerrctr_len "-- expected RX packet length"; rxofctr "RX overflow - core_rxofctr"; rxbadctr "RX bad - core_rxbadctr"; rxvldctr "RX valid cycle - core_rxvldctr"; rxeofctr "RX eof - core_rxeofctr"; rxsnaplen "RX snapshot length"; rxsrcip "RX snapshot - include source IPs"; rxdstip "RX snapshot - include destination IPs"
      mask help: This block sends and receives UDP frames (packets). It accepts a 256 bit wide data stream with user-determined frame breaks. The data stream is wrapped in a UDP frame for transmission. Incoming UDP packets are unwrapped and the data presented as a 256 bit wide stream.
      mask init:
      | temp = eval(get_param(gcb, 'debug_ctr_width'));
      | if temp <= 0,
      |     error('Debug counters cannot be <= zero.');
      | end
      | forty_gbe_mask(gcb)
      settings: AttributesFormatString=incoming_latency=0
      mask TypeOptions flavour: sfp+ | cx4
      mask Callback flavour: forty_gbe_callback
      mask TypeOptions slot: 0 | 1
      mask TypeOptions port_r1: 0 | 1 | 2 | 3
      mask TypeOptions port_r2_cx4: 0 | 1 | 2
      mask TypeOptions port_r2_sfpp: 0 | 1 | 2 | 3
      mask TypeOptions port: 0 | 1 | 2 | 3
      mask Callback show_param: forty_gbe_callback
      mask TypeOptions pre_emph_r2: 0.15 | 0.3 | 0.45 | 0.61 | 0.74 | 0.91 | 1.07 | 1.25 | 1.36 | 1.55 | 1.74 | 1.94 | 2.11 | 2.32 | 2.54 | 2.77
      mask TypeOptions pre_emph: 0 | 1 | 2 | 3
      mask TypeOptions post_emph_r2: 0.18 | 0.19 | 0.2 | 0.39 | 0.63 | 0.82 | 1.07 | 1.32 | 1.6 | 1.65 | 1.94 | 2.21 | 2.52 | 2.76 | 3.08 | 3.41 | 3.77 | 3.97 | 4.36 | 4.73 | 5.16 | 5.47 | 5.93 | 6.38 | 6.89
      mask TypeOptions rxeqmix_r2: 0 | 1 | 2 | 3 | 4 | 5 | 6 | 7
      mask TypeOptions swing_r2: 110 | 210 | 310 | 400 | 480 | 570 | 660 | 740 | 810 | 880 | 940 | 990 | 1040 | 1080 | 1110 | 1130
      mask TypeOptions swing: 400 | 500 | 600 | 700 | 800
      mask Callback debug_en_all:
      | if strcmp(get_param(gcb, 'debug_en_all'), 'on')
      |     set_param(gcb, 'debug_dis_all', 'off')
      | end
      mask Callback debug_dis_all:
      | if strcmp(get_param(gcb, 'debug_dis_all'), 'on')
      |     set_param(gcb, 'debug_en_all', 'off')
      | end
      mask Callback txerrctr:
      | blk = gcb;
      | mask_visibilities = get_param(blk, 'MaskVisibilities');
      | mask_names = get_param(blk, 'MaskNames');
      | if strcmp(get_param(blk, 'txerrctr'), 'on')
      |     mask_visibilities{ismember(mask_names, 'txerrctr_len')} = 'on';
      | else
      |     mask_visibilities{ismember(mask_names, 'txerrctr_len')} = 'off';
      | end
      | set_param(blk, 'MaskVisibilities', mask_visibilities);
      mask TypeOptions txsnaplen: 0 - no snap | 256 | 512 | 1024 | 2048 | 4096 | 8192 | 16384
      mask Callback rxerrctr:
      | blk = gcb;
      | mask_visibilities = get_param(blk, 'MaskVisibilities');
      | mask_names = get_param(blk, 'MaskNames');
      | if strcmp(get_param(blk, 'rxerrctr'), 'on')
      |     mask_visibilities{ismember(mask_names, 'rxerrctr_len')} = 'on';
      | else
      |     mask_visibilities{ismember(mask_names, 'rxerrctr_len')} = 'off';
      | end
      | set_param(blk, 'MaskVisibilities', mask_visibilities);
      mask TypeOptions rxsnaplen: 0 - no snap | 256 | 512 | 1024 | 2048 | 4096 | 8192 | 16384
      mask DialogControl ParameterTabVar0 Prompt: Core
      mask DialogControl ParameterTabVar01 Prompt: Debug counters
      mask DialogControl Control2 Prompt: -------------------------------------
      mask DialogControl Control2_copy Prompt: -------------------------------------
  pipeline1 : Subsystem  AncestorBlock=casper_library_delays/pipeline  mask(pipeline){csp_latency=3}
      mask prompts: csp_latency "Latency"
      mask help:
      | An explicitly laid-out delay line to avoid mapping to SRL16s
      | for use in pipelining to help achieve timing closure.
      mask init:
      | pipeline_init(gcb,'latency',csp_latency);
      settings: AttributesFormatString=Latency = %<latency>
      mask Display:
      | port_label('input', 1, 'd');
      | port_label('output', 1, 'q');
      | disp(['Z^-', num2str(csp_latency)]);
  pipeline2 : Subsystem  AncestorBlock=casper_library_delays/pipeline  mask(pipeline){csp_latency=3}
      mask prompts: csp_latency "Latency"
      mask help:
      | An explicitly laid-out delay line to avoid mapping to SRL16s
      | for use in pipelining to help achieve timing closure.
      mask init:
      | pipeline_init(gcb,'latency',csp_latency);
      settings: AttributesFormatString=Latency = %<latency>
      mask Display:
      | port_label('input', 1, 'd');
      | port_label('output', 1, 'q');
      | disp(['Z^-', num2str(csp_latency)]);
  pipeline3 : Subsystem  AncestorBlock=casper_library_delays/pipeline  mask(pipeline){csp_latency=3}
      mask prompts: csp_latency "Latency"
      mask help:
      | An explicitly laid-out delay line to avoid mapping to SRL16s
      | for use in pipelining to help achieve timing closure.
      mask init:
      | pipeline_init(gcb,'latency',csp_latency);
      settings: AttributesFormatString=Latency = %<latency>
      mask Display:
      | port_label('input', 1, 'd');
      | port_label('output', 1, 'q');
      | disp(['Z^-', num2str(csp_latency)]);
  pipeline4 : Subsystem  AncestorBlock=casper_library_delays/pipeline  mask(pipeline){csp_latency=3}
      mask prompts: csp_latency "Latency"
      mask help:
      | An explicitly laid-out delay line to avoid mapping to SRL16s
      | for use in pipelining to help achieve timing closure.
      mask init:
      | pipeline_init(gcb,'latency',csp_latency);
      settings: AttributesFormatString=Latency = %<latency>
      mask Display:
      | port_label('input', 1, 'd');
      | port_label('output', 1, 'q');
      | disp(['Z^-', num2str(csp_latency)]);
  pipeline5 : Subsystem  AncestorBlock=casper_library_delays/pipeline  mask(pipeline){csp_latency=3}
      mask prompts: csp_latency "Latency"
      mask help:
      | An explicitly laid-out delay line to avoid mapping to SRL16s
      | for use in pipelining to help achieve timing closure.
      mask init:
      | pipeline_init(gcb,'latency',csp_latency);
      settings: AttributesFormatString=Latency = %<latency>
      mask Display:
      | port_label('input', 1, 'd');
      | port_label('output', 1, 'q');
      | disp(['Z^-', num2str(csp_latency)]);
  pipeline6 : Subsystem  AncestorBlock=casper_library_delays/pipeline  mask(pipeline){csp_latency=3}
      mask prompts: csp_latency "Latency"
      mask help:
      | An explicitly laid-out delay line to avoid mapping to SRL16s
      | for use in pipelining to help achieve timing closure.
      mask init:
      | pipeline_init(gcb,'latency',csp_latency);
      settings: AttributesFormatString=Latency = %<latency>
      mask Display:
      | port_label('input', 1, 'd');
      | port_label('output', 1, 'q');
      | disp(['Z^-', num2str(csp_latency)]);
  pipeline7 : Subsystem  AncestorBlock=casper_library_delays/pipeline  mask(pipeline){csp_latency=3}
      mask prompts: csp_latency "Latency"
      mask help:
      | An explicitly laid-out delay line to avoid mapping to SRL16s
      | for use in pipelining to help achieve timing closure.
      mask init:
      | pipeline_init(gcb,'latency',csp_latency);
      settings: AttributesFormatString=Latency = %<latency>
      mask Display:
      | port_label('input', 1, 'd');
      | port_label('output', 1, 'q');
      | disp(['Z^-', num2str(csp_latency)]);
  pipeline8 : Subsystem  AncestorBlock=casper_library_delays/pipeline  mask(pipeline){csp_latency=3}
      mask prompts: csp_latency "Latency"
      mask help:
      | An explicitly laid-out delay line to avoid mapping to SRL16s
      | for use in pipelining to help achieve timing closure.
      mask init:
      | pipeline_init(gcb,'latency',csp_latency);
      settings: AttributesFormatString=Latency = %<latency>
      mask Display:
      | port_label('input', 1, 'd');
      | port_label('output', 1, 'q');
      | disp(['Z^-', num2str(csp_latency)]);
  pipeline9 : Subsystem  AncestorBlock=casper_library_delays/pipeline  mask(pipeline){csp_latency=3}
      mask prompts: csp_latency "Latency"
      mask help:
      | An explicitly laid-out delay line to avoid mapping to SRL16s
      | for use in pipelining to help achieve timing closure.
      mask init:
      | pipeline_init(gcb,'latency',csp_latency);
      settings: AttributesFormatString=Latency = %<latency>
      mask Display:
      | port_label('input', 1, 'd');
      | port_label('output', 1, 'q');
      | disp(['Z^-', num2str(csp_latency)]);
  wires:
  forty_gbe/12(rx_overrun) -> [gbe_sw_rx_orun]
  vld/1 -> Logical/1
  ctrl/1(in_reg) -> Slice4/1, Slice3/1, Slice1/1, Slice/1
  Slice/1 -> [gbe_sw_rst]
  Slice1/1 -> [gbe_sw_en]
  Slice3/1 -> [gbe_stat_rst]
  forty_gbe/5(tx_overflow) -> [gbe_sw_tx_oflow]
  forty_gbe/4(tx_afull) -> [gbe_sw_tx_afull]
  forty_gbe/3(led_tx) -> [gbe_sw_led_tx]
  forty_gbe/2(led_rx) -> [gbe_sw_led_rx]
  forty_gbe/1(led_up) -> [gbe_sw_led_up]
  forty_gbe/11(rx_bad_frame) -> [gbe_sw_rx_bfr]
  Constant/1 -> pipeline2/1(d)
  [gbe_sw_en] -> Register/1
  Register/1 -> Logical/2
  Slice4/1 -> [force_en]
  Logical1/1 -> Register/2
  [force_en] -> Logical1/1
  data/1 -> Delay5/1
  Logical/1 -> Delay6/1
  dest_ip/1 -> Delay7/1
  port/1 -> Delay8/1
  eof/1 -> Delay9/1, Logical1/2
  Constant1/1 -> pipeline1/1(d)
  Delay6/1 -> pipeline7/1(d)
  Delay9/1 -> pipeline3/1(d)
  Delay8/1 -> pipeline4/1(d)
  Delay5/1 -> pipeline8/1(d)
  Delay7/1 -> pipeline5/1(d)
  Delay10/1 -> pipeline6/1(d)
  Delay11/1 -> pipeline9/1(d)
  [gbe_stat_rst] -> Delay10/1
  [gbe_sw_rst] -> Delay11/1
  pipeline6/1(q) -> forty_gbe/9(debug_rst)
  pipeline1/1(q) -> forty_gbe/8(rx_overrun_ack)
  pipeline2/1(q) -> forty_gbe/7(rx_ack)
  pipeline3/1(q) -> forty_gbe/6(tx_end_of_frame)
  pipeline4/1(q) -> forty_gbe/5(tx_dest_port)
  pipeline5/1(q) -> forty_gbe/4(tx_dest_ip)
  pipeline7/1(q) -> forty_gbe/3(tx_valid)
  pipeline8/1(q) -> forty_gbe/2(tx_data)
  pipeline9/1(q) -> forty_gbe/1(rst)
